simulink model "controlador"  (R2021b)
settings: Solver=VariableStepAuto  StartTime=0.0  StopTime=2.5  RelTol=1e-3
undefined symbols (not defined in the file or in its folder): Bm, G, Jt, Kd, Kdp, Kff, Ki, Kip, Km, Kp, Kpp, tau_g, Tmax, Ts
settings Model: Creator=Aluno  LastModifiedBy=Aluno

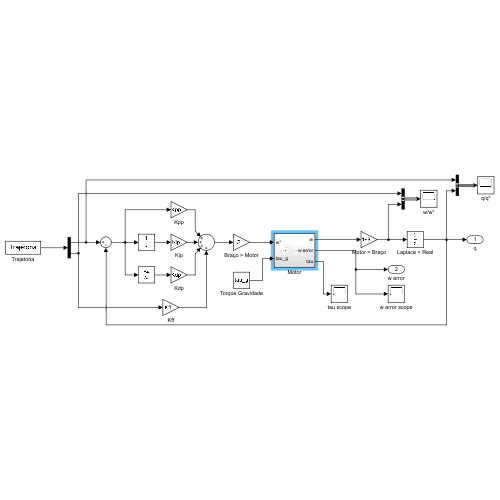
[thumbnail: Simulink's stored preview of the top-level diagram]
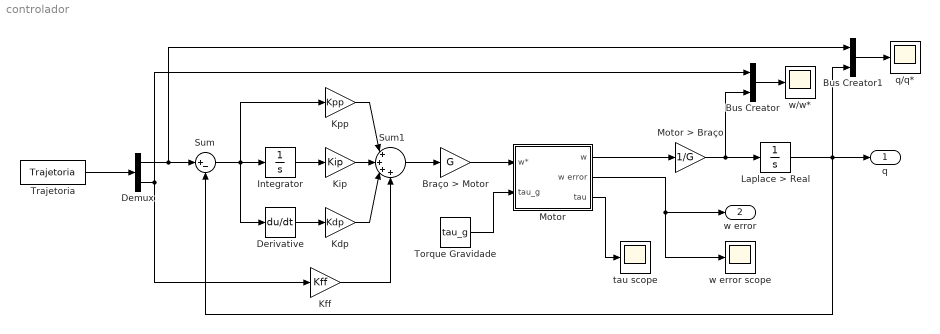
== system controlador ==
  Braço > Motor : Gain  Gain=G
  Bus Creator : BusCreator  Inputs=2
  Bus Creator1 : BusCreator  Inputs=2
  Demux : Demux  Outputs=2
  Derivative : Derivative
  Integrator : Integrator
  Kdp : Gain  Gain=Kdp
  Kff : Gain  Gain=Kff
  Kip : Gain  Gain=Kip
  Kpp : Gain  Gain=Kpp
  Laplace > Real : Integrator
  Motor : Subsystem
  Motor > Braço : Gain  Gain=1/G
  Sum : Sum  Inputs=|+-
  Sum1 : Sum  Inputs=|++++
  Torque Gravidade : Constant  Value=tau_g
  Trajetoria : FromWorkspace  VariableName=Trajetoria
  q/q* : Scope
  tau scope : Scope
  w error scope : Scope
  w/w* : Scope
  q : Outport
  w error : Outport  Port=2
  wires:
  Motor/1(w) -> Motor > Braço/1
  Motor/2(w error) -> w error scope/1, w error/1
  Bus Creator/1 -> w/w*/1
  Motor/3(tau) -> tau scope/1
  Torque Gravidade/1 -> Motor/2(tau_g)
  Motor > Braço/1 -> Bus Creator/2, Laplace > Real/1
  Laplace > Real/1 -> Bus Creator1/2, Sum/2, q/1
  Braço > Motor/1 -> Motor/1(w*)
  Sum/1 -> Derivative/1, Integrator/1, Kpp/1
  Kpp/1 -> Sum1/1
  Sum1/1 -> Braço > Motor/1
  Integrator/1 -> Kip/1
  Trajetoria/1 -> Demux/1
  Demux/1 -> Bus Creator1/1, Sum/1
  Bus Creator1/1 -> q/q*/1
  Demux/2 -> Kff/1, Bus Creator/1
  Kip/1 -> Sum1/2
  Kff/1 -> Sum1/4
  Kdp/1 -> Sum1/3
  Derivative/1 -> Kdp/1

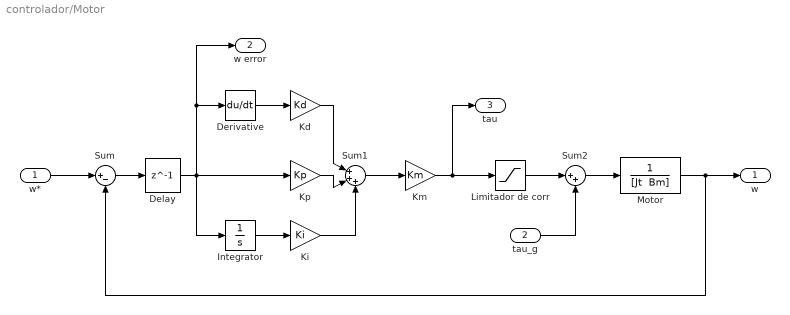
== system controlador/Motor ==
  w* : Inport
  tau_g : Inport  Port=2
  Delay : Delay  DelayLength=1  InitialCondition=0  SampleTime=Ts
  Derivative : Derivative
  Integrator : Integrator
  Kd : Gain  Gain=Kd
  Ki : Gain  Gain=Ki
  Km : Gain  Gain=Km
  Kp : Gain  Gain=Kp
  Limitador de corr : Saturate  UpperLimit=Tmax  LowerLimit=-Tmax
  Motor : TransferFcn  Denominator="[Jt  Bm]"
  Sum : Sum  Inputs=|+-
  Sum1 : Sum  Inputs=|+++
  Sum2 : Sum  Inputs=|++
  w : Outport
  w error : Outport  Port=2
  tau : Outport  Port=3
  wires:
  w*/1 -> Sum/1
  Motor/1 -> w/1, Sum/2
  Integrator/1 -> Ki/1
  Delay/1 -> Integrator/1, Derivative/1, w error/1, Kp/1
  Sum/1 -> Delay/1
  Sum1/1 -> Km/1
  Km/1 -> tau/1, Limitador de corr/1
  Limitador de corr/1 -> Sum2/1
  Sum2/1 -> Motor/1
  tau_g/1 -> Sum2/2
  Ki/1 -> Sum1/3
  Kp/1 -> Sum1/2
  Derivative/1 -> Kd/1
  Kd/1 -> Sum1/1
